simulink model "MA_Zustandsautomat1"  (R2019b)
settings: Solver=VariableStepAuto  StartTime=0.0  StopTime=30  RelTol=1e-3
libraries: simulink x2, dspsigops x1
settings Model: Creator=z004460b  LastModifiedBy=z004460b
settings SFSimCC: CustomCodeUndefinedFunction=UseInterfaceOnly

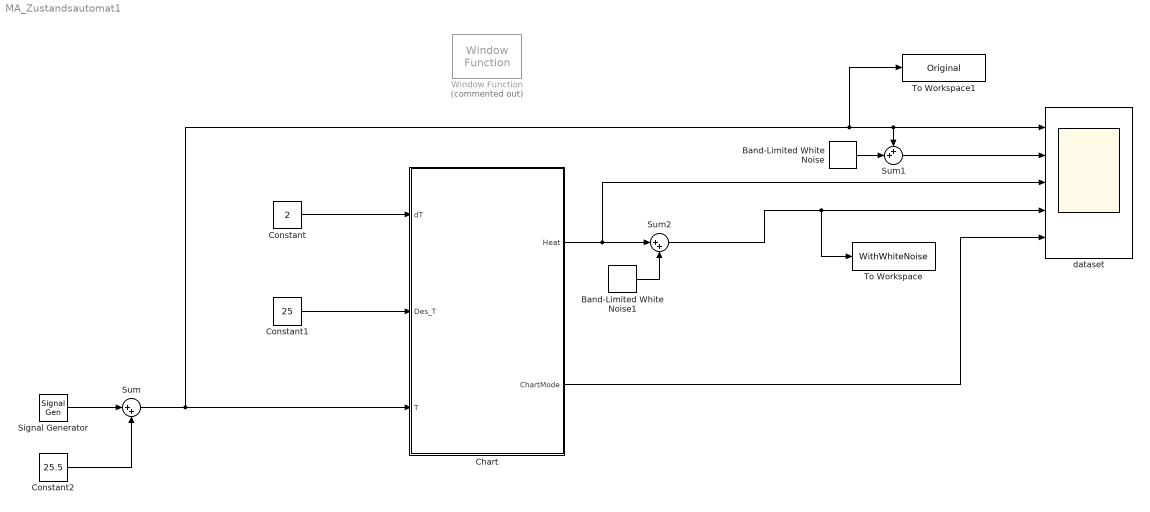
== system MA_Zustandsautomat1 ==
  Band-Limited White Noise : simulink/Sources/Band-Limited White Noise  Cov=[0.1]  Ts=0.1  seed=[23341]
  Band-Limited White Noise1 : simulink/Sources/Band-Limited White Noise  Cov=[0.1]  Ts=0.1  seed=[2341]
  Chart : Stateflow chart  BlockKeywords=__PRM__SERIALIZED__DATA__:Stateflow Chart,Stateflow Diagram  TreatAsAtomicUnit=on
  Constant : Constant  Value=2
  Constant1 : Constant  Value=25
  Constant2 : Constant  Value=25.5
  Signal Generator : SignalGenerator  Amplitude=4.5  Frequency=0.5  Units=rad/sec
  Sum : Sum  Inputs=|++
  Sum1 : Sum  Inputs=++|
  Sum2 : Sum  Inputs=|++
  To Workspace : ToWorkspace  VariableName=WithWhiteNoise  SaveFormat=Timeseries  SampleTime=-1
  To Workspace1 : ToWorkspace  VariableName=Original  SaveFormat=Timeseries  SampleTime=-1
  Window Function : dspsigops/Window Function  Commented=on  winmode=Generate and apply window  wintype=Hamming  sampmode=Continuous  samptime=1  N=64  Rs=50  beta=10  winsamp=Symmetric  UserWindow=hamming  OptParams=off  UserParams={'symmetric'}  dataType=double  isSigned=on  wordLen=16  udDataType=sfix(16)  fracBitsMode=Best precision  numFracBits=15  firstCoeffMode=Binary point scaling  firstCoeffWordLength=8  firstCoeffFracLength=0  prodOutputMode=Slope and bias scaling  prodOutputWordLength=16  prodOutputFracLength=15  roundingMode=Floor  overflowMode=off  numSidelobes=4  sidelobeLevel=-30
      settings: SourceProductName=DSP System Toolbox  SourceProductBaseCode=DS  LockScale=on
  dataset : Scope  NumInputPorts=5
  wires:
  Constant/1 -> Chart/1(dT)
  Constant1/1 -> Chart/2(Des_T)
  Signal Generator/1 -> Sum/1
  Constant2/1 -> Sum/2
  Sum2/1 -> To Workspace/1, dataset/4
  Chart/2(ChartMode) -> dataset/5
  Band-Limited White Noise1/1 -> Sum2/2
  Chart/1(Heat) -> dataset/3, Sum2/1
  Band-Limited White Noise/1 -> Sum1/2
  Sum/1 -> To Workspace1/1, Sum1/1, dataset/1, Chart/3(T)
  Sum1/1 -> dataset/2

== stateflow chart MA_Zustandsautomat1/Chart ==
  state Off
    entry:
    Heat = 0;
  state CoolerOn
    entry:
    Heat = -1;
  state HeaterOn
    entry:
    Heat = 1;
  (default) -> (junction 15)
  (junction 15) -> HeaterOn [order 2] : [T < (Des_T - dT)]
  (junction 15) -> CoolerOn [order 1] : [T > (Des_T + dT)]
  (junction 15) -> Off [order 3]
  Off -> HeaterOn [order 1] : [T < (Des_T - dT)]
  CoolerOn -> Off : [T <= (Des_T + dT)]
  Off -> CoolerOn [order 2] : [T > (Des_T + dT)]
  HeaterOn -> Off : [T >= (Des_T - dT)]
  data: dT input; Des_T input; T input; Heat output; ChartMode output Enum: ChartModeType
